simulink model "SIM_ADCS"  (R2026a)
settings: Solver=ode4  StopTime=sim_time  FixedStep=SIM_dt
InitFcn:
  | hw_ADCS;
undefined symbols (not defined in the file): D2R, K_bdot, Max_dipole, q0_eci2brf, R_E
libraries: matrix_library x2
settings Model: Creator=User  LastModifiedBy=User

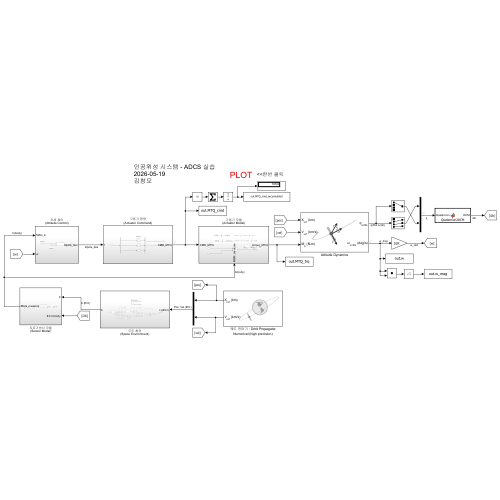
[thumbnail: Simulink's stored preview of the top-level diagram]
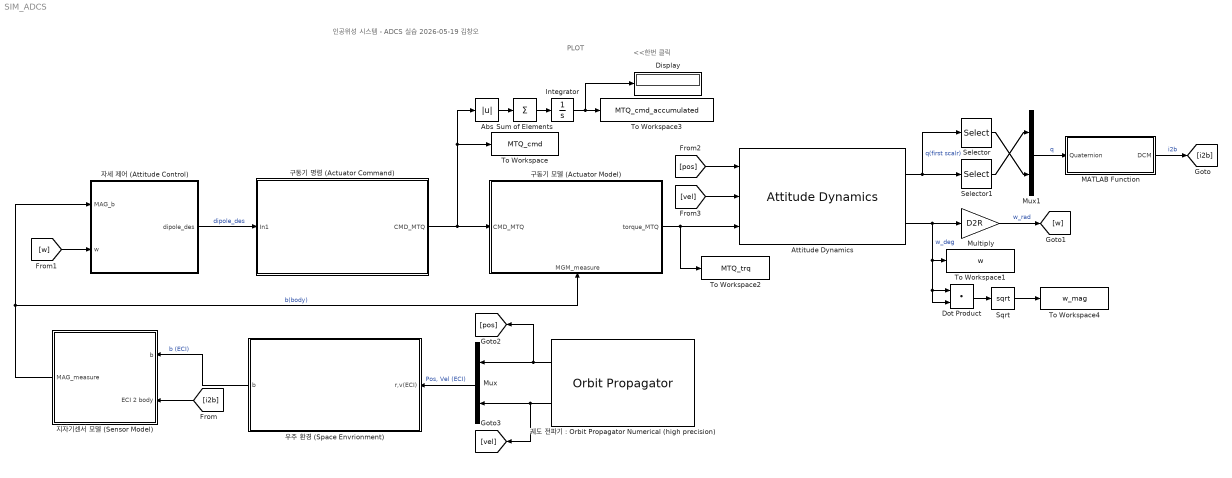
== system SIM_ADCS ==
  note: <<한번 클릭
  note: PLOT
  note: 인공위성 시스템 - ADCS 실습
      | 2026-05-19
      | 김창오
  Abs : Abs  SaturateOnIntegerOverflow=off
  Attitude Dynamics : AttitudeDynamics  startDate=startdate  dateOut=off  inertia=J  attitude=[q0_eci2brf(4) ; q0_eci2brf(1:3)]  attitudeRate=w_b_i2b  useGravGrad=off  units=Metric (km/s)
  Display : Display
  Dot Product : DotProduct  OutDataTypeStr=Inherit: Inherit via internal rule
  Integrator : Integrator
  MATLAB Function : MATLAB Function  TreatAsAtomicUnit=on
  Multiply : Gain  Gain=D2R
  Mux : Mux  Inputs=2
  Mux1 : Mux  Inputs=2
  Selector : Selector  InputPortWidth=4  IndexOptions=Index vector (dialog)  Indices=[1]  OutputSizes=1
  Selector1 : Selector  InputPortWidth=4  IndexOptions=Index vector (dialog)  Indices=[2:4]  OutputSizes=1
  Sqrt : Sqrt
  Sum of Elements : Sum  Inputs=+
  To Workspace : ToWorkspace  VariableName=MTQ_cmd  SampleTime=-1
      settings: Save2DSignal=2-D array (concatenate along first dimension)
  To Workspace1 : ToWorkspace  VariableName=w  SampleTime=-1
      settings: Save2DSignal=2-D array (concatenate along first dimension)
  To Workspace2 : ToWorkspace  VariableName=MTQ_trq  SampleTime=-1
      settings: Save2DSignal=2-D array (concatenate along first dimension)
  To Workspace3 : ToWorkspace  VariableName=MTQ_cmd_accumulated  SampleTime=-1
      settings: Save2DSignal=2-D array (concatenate along first dimension)
  To Workspace4 : ToWorkspace  VariableName=w_mag  SampleTime=-1
      settings: Save2DSignal=2-D array (concatenate along first dimension)
  구동기 명령 (Actuator Command) : Subsystem
  구동기 모델 (Actuator Model) : Subsystem
      settings: PortSchema="{\"entries\":[{\"content\":{\"sides\":[{\"content\":{\"connectorIds\":[\"In1\"]},\"type\":\"ConnectorPlacement.EquallySpacedRectSide\",\"uuid\":\"9a5d12c5-b502-4525-a023-7ee99a1255a7\"},{\"content\":{\"connectorIds\":[\"Out1\"],\"side\":\"RIGHT\"},\"type\":\"ConnectorPlacement.EquallySpacedRectSide\",\"uuid\":\"cfcf6749-1da1-4c6b-830b-5ac0a43c8829\"},{\"content\":{\"side\":\"TOP\"},\"type\":\"ConnectorPlacement.EquallySpacedRectSide\",\"uuid\":\"5cb3e3d5-522e-427f-8524-ebb24c2a230b\"},{\"content\":{\"connectorIds\":[\"In2\"],\"side\":\"BOTTOM\"},\"type\":\"ConnectorPlacement.EquallySpacedRectSide\",\"uuid\":\"ac870c70-2b87-4e53-8b36-c4ab6e5dd940\"}]},\"type\":\"ConnectorPlacement.EquallySpacedConnector\",\"uuid\":\"c00ccf6f-df06-489a-8918-39f520918a65\"}],\"packageUris\":[\"http://schema.mathworks.com/mf0/Connector/R2020b\"],\"version\":\"1.0\"}"
  "궤도 전파기 : Orbit Propagator Numerical (high precision)" : OrbitPropagator  startDate=startdate  dateOut=off  stateFormatNum=ICRF state vector  stateFormatKep=ICRF state vector  inertialPosition=r0_eci  inertialVelocity=v0_eci  fixedPosition=[-4142689.0 -2676864.7 -4669861.6]  fixedVelocity=[1452.7 -6720.7 2568.1]  customR=3396200  customMu=4.305e13  customJ2=1.0826269e-03  customOmega=4.06125949e-3  outputTransform=on  units=Metric (km/s)
  우주 환경 (Space Envrionment) : Subsystem
  자세 제어 (Attitude Control) : Subsystem
  지자기센서 모델 (Sensor Model) : Subsystem
  wires:
  Mux/1 -> 우주 환경 (Space Envrionment)/1(r,v(ECI))  "Pos, Vel (ECI)"
  자세 제어 (Attitude Control)/1(dipole_des) -> 구동기 명령 (Actuator Command)/1(In1)  "dipole_des"
  구동기 모델 (Actuator Model)/1(torque_MTQ) -> To Workspace2/1, Attitude Dynamics/3
  우주 환경 (Space Envrionment)/1(b) -> 지자기센서 모델 (Sensor Model)/1(b)  "b (ECI)"
  [i2b] -> 지자기센서 모델 (Sensor Model)/2(ECI 2 body)
  지자기센서 모델 (Sensor Model)/1(MAG_measure) -> 구동기 모델 (Actuator Model)/2(MGM_measure), 자세 제어 (Attitude Control)/1(MAG_b)  "b(body)"
  구동기 명령 (Actuator Command)/1(CMD_MTQ) -> To Workspace/1, Abs/1, 구동기 모델 (Actuator Model)/1(CMD_MTQ)
  [w] -> 자세 제어 (Attitude Control)/2(w)
  "궤도 전파기 : Orbit Propagator Numerical (high precision)"/2 -> [vel], Mux/2
  "궤도 전파기 : Orbit Propagator Numerical (high precision)"/1 -> [pos], Mux/1
  Attitude Dynamics/1 -> Selector/1, Selector1/1  "q(first scalr)"
  Attitude Dynamics/2 -> To Workspace1/1, Dot Product/1, Dot Product/2, Multiply/1  "w_deg"
  Mux1/1 -> MATLAB Function/1(Quaternion)  "q"
  [pos] -> Attitude Dynamics/1
  [vel] -> Attitude Dynamics/2
  Selector/1 -> Mux1/2
  Selector1/1 -> Mux1/1
  MATLAB Function/1(DCM) -> [i2b]  "i2b"
  Multiply/1 -> [w]  "w_rad"
  Abs/1 -> Sum of Elements/1
  Sum of Elements/1 -> Integrator/1
  Integrator/1 -> Display/1, To Workspace3/1
  Dot Product/1 -> Sqrt/1
  Sqrt/1 -> To Workspace4/1

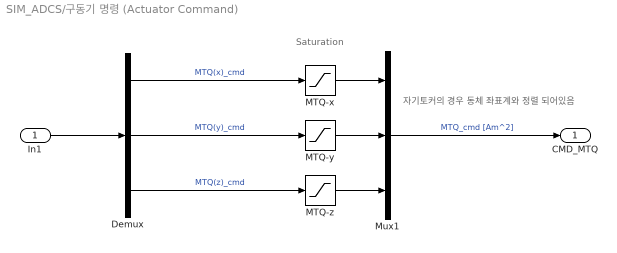
== system SIM_ADCS/구동기 명령 (Actuator Command) ==
  note: 자기토커의 경우 동체 좌표계와 정렬 되어있음
  note: Saturation
  In1 : Inport
  Demux : Demux  Outputs=3
  MTQ-x : Saturate  UpperLimit=Max_dipole  LowerLimit=-Max_dipole
  MTQ-y : Saturate  UpperLimit=Max_dipole  LowerLimit=-Max_dipole
  MTQ-z : Saturate  UpperLimit=Max_dipole  LowerLimit=-Max_dipole
  Mux1 : Mux  Inputs=3
  CMD_MTQ : Outport
  wires:
  Mux1/1 -> CMD_MTQ/1  "MTQ_cmd [Am^2]"
  MTQ-y/1 -> Mux1/2
  MTQ-x/1 -> Mux1/1
  MTQ-z/1 -> Mux1/3
  Demux/3 -> MTQ-z/1  "MTQ(z)_cmd"
  Demux/2 -> MTQ-y/1  "MTQ(y)_cmd"
  Demux/1 -> MTQ-x/1  "MTQ(x)_cmd"
  In1/1 -> Demux/1

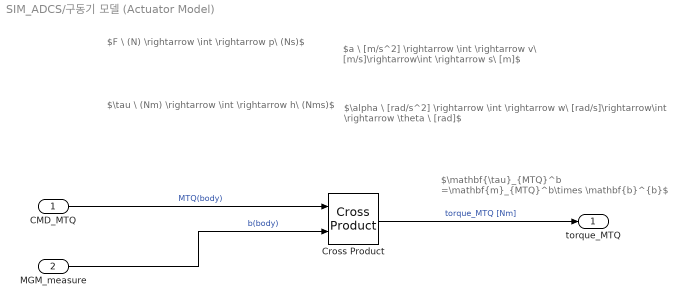
== system SIM_ADCS/구동기 모델 (Actuator Model) ==
  note: $\mathbf{\tau}_{MTQ}^b =\mathbf{m}_{MTQ}^b\times \mathbf{b}^{b}$
  note: $\alpha \ [rad/s^2] \rightarrow \int \rightarrow w\ [rad/s]\rightarrow\int \rightarrow \theta \ [rad]$
  note: $a \ [m/s^2] \rightarrow \int \rightarrow v\ [m/s]\rightarrow\int \rightarrow s\ [m]$
  note: $\tau \ (Nm) \rightarrow \int \rightarrow h\ (Nms)$
  note: $F \ (N) \rightarrow \int \rightarrow p\ (Ns)$
  CMD_MTQ : Inport
  MGM_measure : Inport  Port=2
  Cross Product : matrix_library/Cross Product
  torque_MTQ : Outport
  wires:
  CMD_MTQ/1 -> Cross Product/1  "MTQ(body)"
  MGM_measure/1 -> Cross Product/2  "b(body)"
  Cross Product/1 -> torque_MTQ/1  "torque_MTQ [Nm]"

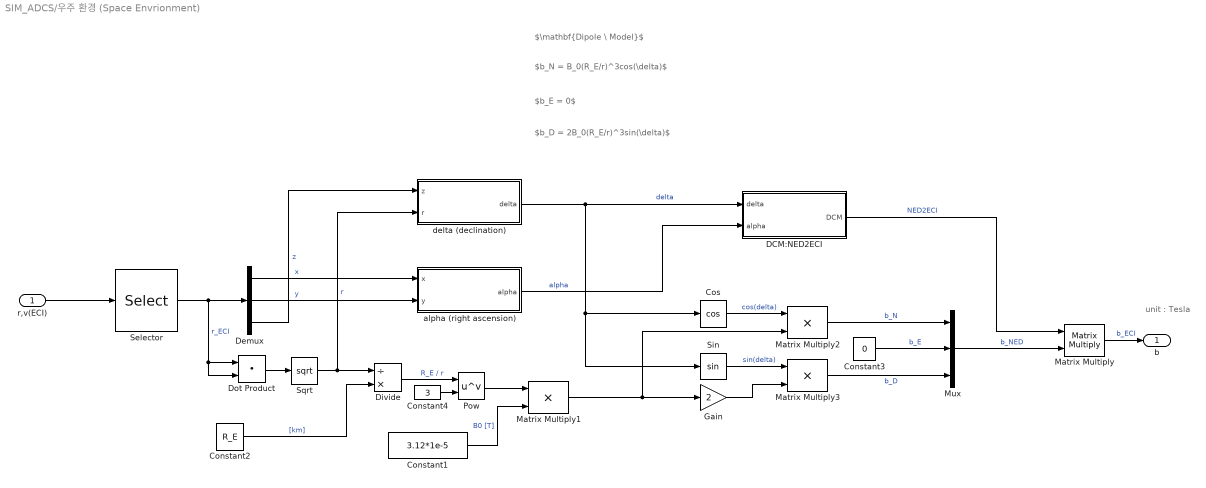
== system SIM_ADCS/우주 환경 (Space Envrionment) ==
  note: unit : Tesla
  note: $b_N = B_0(R_E/r)^3cos(\delta)$
  note: $\mathbf{Dipole \ Model}$
  note: $b_E = 0$
  note: $b_D = 2B_0(R_E/r)^3sin(\delta)$
  r,v(ECI) : Inport
  Constant1 : Constant  Value=3.12*1e-5
  Constant2 : Constant  Value=R_E
  Constant3 : Constant  Value=0
  Constant4 : Constant  Value=3
  Cos : Trigonometry  Operator=cos
  DCM:NED2ECI : Subsystem
  Demux : Demux  Outputs=3
  Divide : Product  Inputs=/*
  Dot Product : DotProduct  OutDataTypeStr=Inherit: Inherit via internal rule
  Gain : Gain  Gain=2
  Matrix Multiply : Product  Multiplication=Matrix(*)
  Matrix Multiply1 : Product
  Matrix Multiply2 : Product
  Matrix Multiply3 : Product
  Mux : Mux  Inputs=3
  Pow : Math  Operator=pow  RndMeth=Zero
  Selector : Selector  InputPortWidth=6  IndexOptions=Index vector (dialog)  Indices=[1 2 3]  OutputSizes=1
  Sin : Trigonometry
  Sqrt : Sqrt
  alpha (right ascension) : Subsystem
  delta (declination) : Subsystem
  b : Outport
  wires:
  r,v(ECI)/1 -> Selector/1
  Mux/1 -> Matrix Multiply/2  "b_NED"
  Matrix Multiply/1 -> b/1  "b_ECI"
  DCM:NED2ECI/1(DCM) -> Matrix Multiply/1  "NED2ECI"
  Constant1/1 -> Matrix Multiply1/2  "B0 [T]"
  Constant2/1 -> Divide/2  "[km]"
  Selector/1 -> Dot Product/2, Dot Product/1, Demux/1  "r_ECI"
  Demux/1 -> alpha (right ascension)/1(x)  "x"
  Demux/2 -> alpha (right ascension)/2(y)  "y"
  Demux/3 -> delta (declination)/1(z)  "z"
  Dot Product/1 -> Sqrt/1
  Constant3/1 -> Mux/2  "b_E"
  Matrix Multiply3/1 -> Mux/3  "b_D"
  Sqrt/1 -> Divide/1, delta (declination)/2(r)  "r"
  delta (declination)/1(delta) -> Sin/1, Cos/1, DCM:NED2ECI/1(delta)  "delta"
  alpha (right ascension)/1(alpha) -> DCM:NED2ECI/2(alpha)  "alpha"
  Constant4/1 -> Pow/2
  Divide/1 -> Pow/1  "R_E / r"
  Pow/1 -> Matrix Multiply1/1
  Matrix Multiply2/1 -> Mux/1  "b_N"
  Cos/1 -> Matrix Multiply2/1  "cos(delta)"
  Matrix Multiply1/1 -> Matrix Multiply2/2, Gain/1
  Sin/1 -> Matrix Multiply3/1  "sin(delta)"
  Gain/1 -> Matrix Multiply3/2

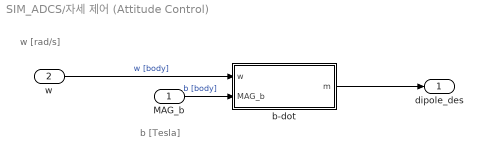
== system SIM_ADCS/자세 제어 (Attitude Control) ==
  note: w [rad/s]
  note: b [Tesla]
  MAG_b : Inport
  w : Inport  Port=2
  b-dot : Subsystem
  dipole_des : Outport
  wires:
  w/1 -> b-dot/1(w)  "w [body]"
  MAG_b/1 -> b-dot/2(MAG_b)  "b [body]"
  b-dot/1(m) -> dipole_des/1

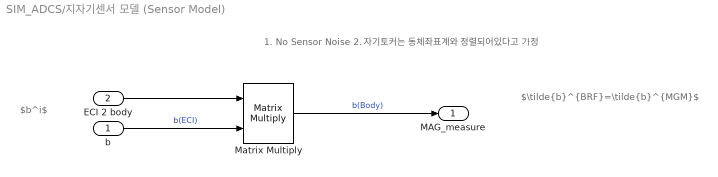
== system SIM_ADCS/지자기센서 모델 (Sensor Model) ==
  note: 1. No Sensor Noise
      | 2. 자기토커는 동체좌표계와 정렬되어있다고 가정
  note: $\tilde{b}^{BRF}=\tilde{b}^{MGM}$
  note: $b^i$
  b : Inport
  ECI 2 body : Inport  Port=2
  Matrix Multiply : Product  Multiplication=Matrix(*)
  MAG_measure : Outport
  wires:
  b/1 -> Matrix Multiply/2  "b(ECI)"
  ECI 2 body/1 -> Matrix Multiply/1
  Matrix Multiply/1 -> MAG_measure/1  "b(Body)"

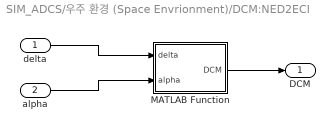
== system SIM_ADCS/우주 환경 (Space Envrionment)/DCM:NED2ECI ==
  delta : Inport
  alpha : Inport  Port=2
  MATLAB Function : MATLAB Function  TreatAsAtomicUnit=on
  DCM : Outport
  wires:
  delta/1 -> MATLAB Function/1(delta)
  alpha/1 -> MATLAB Function/2(alpha)
  MATLAB Function/1(DCM) -> DCM/1

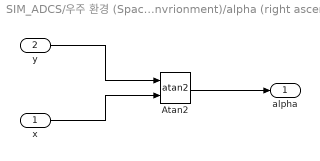
== system SIM_ADCS/우주 환경 (Space Envrionment)/alpha (right ascension) ==
  x : Inport
  y : Inport  Port=2
  Atan2 : Trigonometry  Operator=atan2
  alpha : Outport
  wires:
  y/1 -> Atan2/1
  x/1 -> Atan2/2
  Atan2/1 -> alpha/1

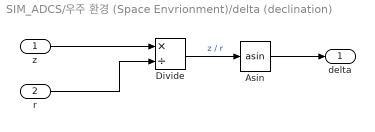
== system SIM_ADCS/우주 환경 (Space Envrionment)/delta (declination) ==
  z : Inport
  r : Inport  Port=2
  Asin : Trigonometry  Operator=asin
  Divide : Product  Inputs=*/
  delta : Outport
  wires:
  z/1 -> Divide/1
  r/1 -> Divide/2
  Divide/1 -> Asin/1  "z / r"
  Asin/1 -> delta/1

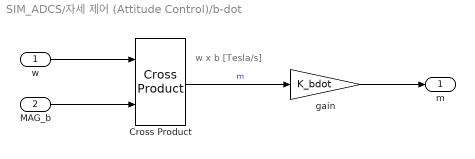
== system SIM_ADCS/자세 제어 (Attitude Control)/b-dot ==
  note: w x b [Tesla/s]
  w : Inport
  MAG_b : Inport  Port=2
  Cross Product : matrix_library/Cross Product
  gain : Gain  Gain=K_bdot
  m : Outport
  wires:
  MAG_b/1 -> Cross Product/2
  w/1 -> Cross Product/1
  Cross Product/1 -> gain/1  "m"
  gain/1 -> m/1

== matlab function SIM_ADCS/MATLAB Function ==
  data: Quaternion input; DCM output
function DCM  = Quaternion2DCM(Quaternion)

q1 = Quaternion(1);
q2 = Quaternion(2);
q3 = Quaternion(3);
q4 = Quaternion(4);

DCM = [q1^2 - q2^2 - q3^2 + q4^2, 2*(q1*q2 + q3*q4), 2*(q1*q3 - q2*q4);
    2*(q1*q2 - q3*q4), -q1^2 + q2^2 - q3^2 + q4^2, 2*(q2*q3+q1*q4);
    2*(q1*q3 + q2*q4), 2*(q2*q3 - q1*q4), -q1^2 - q2^2 + q3^2 + q4^2;];

% qv = [q1; q2; q3;];
% qvX = [0 -q3 q2; q3 0 -q1; -q2 q1 0;];
% C_ = (q4^2 - qv'*qv)*eye(3) + 2*qv*qv' - 2*q4*qvX;

end

== matlab function SIM_ADCS/우주 환경 (Space Envrionment)/DCM:NED2ECI/MATLAB Function ==
  data: delta input; DCM output; alpha input
function DCM = fcn(delta, alpha)

a = alpha;
d = delta;

rot1 = [cos(a) sin(a) 0 ;
       -sin(a) cos(a) 0 ;
       0        0     1 ];
rot2 = [-1  0  0;
         0  1  0;
         0  0 -1];
rot3 = [sin(d) 0 -cos(d) ;
        0      1       0 ;
        cos(d) 0  sin(d) ];

DCM = rot3*rot2*rot1;
